simulink model "customcodetest"  (R2018b)
settings: Solver=FixedStepDiscrete  StartTime=0.0  StopTime=Inf  RelTol=1e-3  EnableMultiTasking=on
undefined symbols (not defined in the file or in its folder): Down, GPTRIP1SEL, GPTRIP2SEL, TZ1, TZ2, Up
libraries: c2000lib x1, c2837xDlib x1, c2802xlib x1
settings Model: ExtModeTrigDuration=8  Creator=ThinkPad  LastModifiedBy=ThinkPad
settings OptimizationCC: DefaultUnderspecifiedDataType=single  EnhancedBackFolding=on  PassReuseOutputArgsAs=Individual arguments  MaxStackSize=512  OptimizeBlockOrder=speed  DifferentSizesBufferReuse=on  OptimizationCustomize=off
settings DebuggingCC: ParameterTunabilityLossMsg=error
settings HardwareCC: ProdBitPerChar=16  ProdBitPerInt=16  ProdBitPerPointer=32  ProdBitPerSizeT=32  ProdBitPerPtrDiffT=32  ProdLargestAtomicInteger=Integer  ProdLargestAtomicFloat=None  ProdWordSize=16  ProdLongLongMode=on  ProdHWDeviceType=Texas Instruments->C2000
settings SFSimCC: MATLABDynamicMemAlloc=off
settings RTWCC: SystemTargetFile=ert.tlc  HardwareBoard=TI Delfino F2837xD  TemplateMakefile=ert_default_tmf  GenerateReport=on  Toolchain=Texas Instruments Code Composer Studio (C2000)  IncludeHyperlinkInReport=on  LaunchReport=on  GenerateTraceInfo=on  GenerateTraceReport=on  GenerateTraceReportSl=on  GenerateTraceReportSf=on  GenerateTraceReportEml=on
settings RTWCC: CustomHeaderCode=|
  | #include "F28x_Project.h"     // Device Headerfile and Examples Include File
  | 
  | #define TEST_PASS 0xABCDABCD
  | #define TEST_FAIL 0xDEADDEAD
  | 
  | 
  | Uint16    *ExRamStart = (Uint16 *)0x300000;
  | extern void setup_emif1_pinmux_async_16bit(Uint16);
  | #define EMIF1 0
  | #define EMIF2 1
  | 
  | #define MEM_D_WIDTH 		1 			// 16Bit Memory Interface
  | #define TURN_AROUND_TIME 	0			// Turn Around time of 2 Emif Clock
  | #define RD_SETUP_TIME 		0			// Read Setup time of 1 Emif Clock
  | #define RD_STROBE_TIME 		3			// Read Strobe time of 4 Emif Clock
  | #define RD_HOLD_TIME 		0			// Read Hold time of 1 Emif Clock
  | #define WR_SETUP_TIME 		0			// Write Hold time of 1 Emif Clock
  | #define WR_STROBE_TIME 		0			// Write Setup time of 1 Emif Clock
  | #define WR_HOLD_TIME 		0			// Write Hold time of 1 Emif Clock
  | #define EXTEND_WAIT 		0			// Disable Extended Wait
  | #define STROBE_SEL 			0			// Disable Strobe Mode.
  | #define WAIT_POLAR_INV 		0
  | #define WAIT_COUNT 			0
  | 
  | 
  | Uint16  ErrCount = 0;
  | Uint32  TEST_STATUS;
  | int i;
settings RTWCC: CustomInitializer=|
  | char ErrCount_local;
  | 	TEST_STATUS = TEST_FAIL;
  | 
  | 	InitSysCtrl();
  | 
  |  	DINT;
  | 
  | //  Initialize the PIE control registers to their default state.
  | //  The default state is all PIE interrupts disabled and flags
  | //  are cleared.
  | //  This function is found in the F2837xS_PieCtrl.c file.
  |     InitPieCtrl();
  | 
  | // Disable CPU interrupts and clear all CPU interrupt flags:
  |         EALLOW;
  | 	IER = 0x0000;
  | 	IFR = 0x0000;
  | 	EDIS;
  | 
  | // Initialize the PIE vector table with pointers to the shell Interrupt
  | // GService Routines (ISR).
  | // This will populate the entire table, even if the interrupt
  | // is not used in this example.  This is useful for debug purposes.
  | // The shell ISR routines are found in F2837xS_DefaultIsr.c.
  | // This function is found in F2837xS_PieVect.c.
  |    InitPieVectTable();
  | 
  | //Configure to run EMIF1 on full Rate (EMIF1CLK = CPU1SYSCLK)
  |   EALLOW;
  |   ClkCfgRegs.PERCLKDIVSEL.bit.EMIF1CLKDIV = 0x0;
  |   EDIS;
  | 
  |   EALLOW;
  | 
  | //Disable Access Protection (CPU_FETCH/CPU_WR/DMA_WR)
  |   Emif1ConfigRegs.EMIF1ACCPROT0.all = 0x0;
  |   if (Emif1ConfigRegs.EMIF1ACCPROT0.all != 0x0)
  |   {
  |       ErrCount++;
  |   }
  | 
  | // Commit the configuration related to protection. Till this bit remains set
  | // content of EMIF1ACCPROT0 register can't be changed.
  |   Emif1ConfigRegs.EMIF1COMMIT.all = 0x1;
  |   if(Emif1ConfigRegs.EMIF1COMMIT.all != 0x1)
  |   {
  | 	 ErrCount++;
  |   }
  | 
  | // Lock the configuration so that EMIF1COMMIT register can't be changed any more.
  |   Emif1ConfigRegs.EMIF1LOCK.all = 0x1;
  |   if (Emif1ConfigRegs.EMIF1LOCK.all != 1)
  |   {
  | 	  ErrCount++;
  |   }
  | 
  |   EDIS;
  | 
  | //Configure GPIO pins for EMIF1
  |   setup_emif1_pinmux_async_16bit(0);
  | 
  | 
  |   //////////////////////////////////////////////
  |   Uint16 i=0;
  | 	for(i = 0; i < 0xFFFF; i++)
  | 	{
  | 		*(ExRamStart + i) = 0x5555;
  | 		if(*(ExRamStart + i) != 0x5555)
  | 		{
  | 			while(1);
  | 		}
  | 	}
  | 	asm(" ESTOP0");
  | 	for(i = 0; i < 0xFFFF; i++)
  | 	{
  | 		*(ExRamStart + i) = 0xAAAA;
  | 		if(*(ExRamStart + i) != 0xAAAA)
  | 		{
  | 			while(1);
  | 		}
  | 	}
  | 	asm(" ESTOP0");
  | 	for(i = 0; i< 0xFFFF; i++)
  | 	{
  | 		*(ExRamStart + i) = i;
  | 		if(*(ExRamStart + i) != i)
  | 		{
  | 			while(1);
  | 		}
  | 		if(*ExRamStart == 0x4000)
  | 		 {
  |            while(1);
  | 		 }
  | 	}
  | 	asm(" ESTOP0");
  |   while (1);
settings CodeAppCC: ForceParamTrailComments=on  IgnoreCustomStorageClasses=off  OperatorAnnotations=on  SimulinkDataObjDesc=on  SFDataObjDesc=on  InsertBlockDesc=on
settings ERTTargetCC: CodeReplacementLibrary=TI C28x

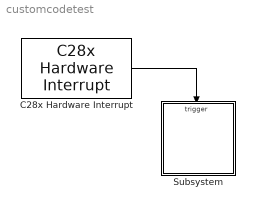
== system customcodetest ==
  C28x Hardware Interrupt : c2000lib/Scheduling/C28x Hardware Interrupt  irqnumbers=[3]  pienumbers=[1]  irqpriorities=[30]  irqpreempts=[0]  showinput=off  dspchiptype=C280X
      settings: SourceProductName=Embedded Coder Support Package for Texas Instruments C2000 Processors  SourceProductBaseCode=TIC2000
  Subsystem : Subsystem
  wires:
  C28x Hardware Interrupt/1 -> Subsystem/Trigger

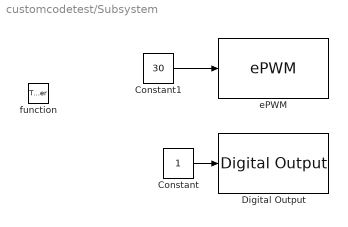
== system customcodetest/Subsystem ==
  function : TriggerPort  TriggerType=function-call  VariantControl=(inherit)  SampleTime=1e-5
  Constant : Constant
  Constant1 : Constant  Value=30
  Digital Output : c2837xDlib/Digital Output  GPIO_Number=GPIO48~GPIO55  GPIO_Bit0=on  GPIO_BIT0_Toggle=off  GPIO_Bit1=off  GPIO_BIT1_Toggle=off  GPIO_Bit2=off  GPIO_BIT2_Toggle=off  GPIO_Bit3=off  GPIO_BIT3_Toggle=on  GPIO_Bit4=off  GPIO_BIT4_Toggle=off  GPIO_Bit5=off  GPIO_BIT5_Toggle=off  GPIO_Bit6=off  GPIO_BIT6_Toggle=off  GPIO_Bit7=off  GPIO_BIT7_Toggle=off
      settings: SourceProductName=Embedded Coder Support Package for Texas Instruments C2000 Processors  SourceProductBaseCode=TIC2000
  ePWM : c2802xlib/ePWM  useModule=ePWM1  ePWMxLINKTBPRD=Not Linked  periodUnits=Clock cycles  timerSource=Specify via dialog  timerPeriod_clk=64000  timerPeriod_sec=0.0001  tbshadow=Counter equals to zero  countingMode=Up-Down  phaseActiveEnable=Disable  phaseDirection=Count down after sync  phaseActive=0  synchronizationEnable=off  dcaevt1Sync=off  dcbevt1Sync=off  synchronizationOption=Disable  clockPrescale=1  HSclockPrescale=1  enswap=off  ePWMxAStatus=on  ePWMxAactionLogic1=Set  ePWMxAactionLogic2=Clear  ePWMxAactionLogic3=Clear  ePWMxAactionLogic4=Set  ePWMxAactionLogic5=Do nothing  ePWMxAactionLogic6=Do nothing  ePWMxALoadMode=Load on counter equals to zero (CTR=Zero)  ePWMxACSFenable=off  ePWMxACSFvalue=Forcing disable  ePWMxASFreload=Zero  ePWMxBStatus=off  ePWMxBactionLogic1=Set  ePWMxBactionLogic2=Clear  ePWMxBactionLogic3=Do nothing  ePWMxBactionLogic4=Do nothing  ePWMxBactionLogic5=Clear  ePWMxBactionLogic6=Set  ePWMxBLoadMode=Load on counter equals to zero (CTR=Zero)  ePWMxBCSFenable=off  ePWMxBCSFvalue=Forcing disable  ePWMxBSFreload=Zero  ePWNxBOutWay=off  ePWMxLINKCMPA=Not Linked  CMPAUnits=Clock cycles  CMPASource=Input port  CMPAValue_per=50  CMPAValue_clk=32000  enCMPAshadow=Counter equals to zero  ePWMxLINKCMPB=Not Linked  CMPBUnits=Clock cycles  CMPBSource=Specify via dialog  CMPBValue_per=50  CMPBValue_clk=32000  enCMPBshadow=Counter equals to zero  ePWMxLINKCMPC=Not Linked  CMPCUnits=Clock cycles  CMPCSource=Specify via dialog  CMPCValue_per=50  CMPCValue_clk=32000  enCMPCshadow=Counter equals to zero  ePWMxLINKCMPD=Not Linked  CMPDUnits=Clock cycles  CMPDSource=Specify via dialog  CMPDValue_per=50  CMPDValue_clk=32000  enCMPDshadow=Counter equals to zero  enableDBePWMxA=off  enableDBePWMxB=off  enhalfcycle=off  DBpolarity=Active high (AH)  DBedgeDelay=Positive  DBSource_ePWMxA=ePWMxA  DBSource_ePWMxB=ePWMxA  DBperiodSource=Specify via dialog  REDperiod=0  FEDperiod=0  adcstartModuleA=off  adcrequestEventA=First event  adcstartEventA=Digital Compare Module A Event 1 start of conversion (DCAEVT1.soc)  adcstartEventA_type2=Digital Compare Module A Event 1 start of conversion (DCAEVT1.soc)  adcstartModuleB=off  adcrequestEventB=First event  adcstartEventB=Counter equals to zero (CTR=Zero)  adcstartEventB_type2=Counter equals to zero (CTR=Zero)  intEn=off  intPrd=First event  intSel=Counter equals to zero (CTR=Zero)  intSel_type2=Counter equals to zero (CTR=Zero)  hrpe=off  enHRPWM=off  HRPWM_LoadMode=Counter equals to period (CTR=PRD)  HRPWM_CTLMode=Duty or Period control mode  HRPWM_EDGMode=Both edge  hrpeb=off  enHRPWMB=off  HRPWM_LoadModeB=Counter equals to zero (CTR=ZERO)  HRPWM_CTLModeB=Duty or Period control mode  HRPWM_EDGModeB=Both edge  enSFO=on  enautoconv=on  chopperEnable=off  chopperFrequency=1  chopperFirstwidth=1  chopperDuty=12.5%  tripZonesource=Specify via dialog  tzselOSHT1=off  tzselOSHT2=off  tzselOSHT3=off  tzselOSHDCAEV1=off  tzselOSHDCBEV1=off  tzselCBC1=off  tzselCBC2=off  tzselCBC3=off  tzselCBCDCAEV2=off  tzselCBCDCBEV2=off  tzselOSHT4=off  tzselOSHT5=off  tzselOSHT6=off  tzselCBC4=off  tzselCBC5=off  tzselCBC6=off  enTzOstIntr=off  enTzCbcIntr=off  enTzDCAEVT1Intr=off  enTzDCAEVT2Intr=off  enTzDCBEVT1Intr=off  enTzDCBEVT2Intr=off  ePWMxAforced=No action  ePWMxBforced=No action  DCAEVT1forced=No action  DCBEVT1forced=No action  DCAEVT2forced=No action  DCBEVT2forced=No action  dcah=Trip Zone 1 input (TZ1)  dcal=Trip Zone 2 input (TZ2)  dcbh=Trip Zone 1 input (TZ1)  dcbl=Trip Zone 2 input (TZ2)  dcah_type2=GPTRIP1SEL/(TZ1)  dcal_type2=GPTRIP2SEL/(TZ2)  dcbh_type2=GPTRIP1SEL/(TZ1)  dcbl_type2=GPTRIP2SEL/(TZ2)  gendcaevt1=Event disabled  gendcaevt2=Event disabled  gendcbevt1=Event disabled  gendcbevt2=Event disabled  dcaevt1src=DCAEVT1 with sync  dcaevt2src=DCAEVT2 with sync  dcbevt1src=DCBEVT1 with sync  dcbevt2src=DCBEVT2 with sync  pulsesel=Counter equals to zero (CTR=Zero)  blankinv=off  blankoffset=0  blankwidth=0  evsrcsel=Filtered version of DCAEVT1 (DCAEVT1FILT)  encape=off  PwmType=C2000_Type4
      settings: SourceProductName=Embedded Coder Support Package for Texas Instruments C2000 Processors
  wires:
  Constant/1 -> Digital Output/1
  Constant1/1 -> ePWM/1
